simulink library "MIL_Test"  (Simulink 7.0)
values from neighbouring files (symbols this model uses):
  TID = min('TI' == AFT(1:2))    [PAS_callback.m]    (also in PSTID_callback.m = [block '/TID'])
undefined symbols (not defined in the file or in its folder): getdatatypespecs, slcm, StepSize
libraries: simulink x71, MIL_Test x6
(part 3 of 11)

== system MIL_Test/Validation Function/TODO/Validation FunctionsTemplate ==
  InOut Bus : Inport  OutDataType=sfix(16)  OutScaling=2^0
  Arbitration : Subsystem
  Bus Creator : BusCreator  Inputs=2
  Bus Creator4 : BusCreator  Inputs=2
  Bus Selector : BusSelector  OutputSignals=signal1.signal1
  Datatype conversion : Subsystem  TreatAsAtomicUnit=on
  Requirement : Subsystem  mask{No=1}
      mask prompts: No "Number of single Validation Functions"
      mask StyleString: popup(1|2|3|4|5|6|7|8|9|10|11|12|13|14|15|16|17|18|19|20)
      mask CallbackString: ReqInVF_callback(gcb);
  Requirement2 : Subsystem  mask{No=1}
      mask prompts: No "Number of single Validation Functions"
      mask StyleString: popup(1|2|3|4|5|6|7|8|9|10|11|12|13|14|15|16|17|18|19|20)
      mask CallbackString: ReqInVF_callback(gcb);
  Terminator : Terminator
  ReqVerdict Bus : Outport  OutDataType=sfix(16)  OutScaling=2^0
  Overall Verdict : Outport  Port=2  OutDataType=sfix(16)  OutScaling=2^0
  wires:
  Bus Selector/1 -> Arbitration/1(In1), Bus Creator4/1  "<signal1>"
  Bus Creator4/1 -> ReqVerdict Bus/1
  Datatype conversion/1(InOut Bus) -> Requirement/1(InOut Bus), Requirement2/1(InOut Bus)
  Arbitration/1(Out1) -> Overall Verdict/1
  Requirement/1(Validation Information) -> Bus Creator/1
  Bus Creator/1 -> Terminator/1, Bus Selector/1
  InOut Bus/1 -> Datatype conversion/1(InOutBus)
  Requirement2/1(Validation Information) -> Bus Creator/2

== system MIL_Test/Validation Function/Test Evaluation Architecture/<system name> ==
  InOut  Bus : Inport  OutDataType=sfix(16)  OutScaling=2^0
  <Requirement name> : Subsystem  Description=Requirement template. Create a new requirement from this template.  mask{No=1}
      mask prompts: No "Number of single Validation Functions"
      mask StyleString: popup(1|2|3|4|5|6|7|8|9|10|11|12|13|14|15|16|17|18|19|20)
      mask CallbackString: ReqName_callback(gcb);
  Arbitration : Subsystem
  Bus Creator : BusCreator  Inputs=1
  Bus Creator1 : BusCreator  Inputs=2
  Bus Creator4 : BusCreator  Inputs=1
  Bus Selector : BusSelector  OutputSignals=signal1.signal1.signal1
  Signal Conversion : SignalConversion  ConversionOutput=Bus copy
  Terminator : Terminator
  Eval Results : Outport  OutDataType=sfix(16)  OutScaling=2^0
  wires:
  Bus Selector/1 -> Bus Creator4/1, Arbitration/1(In1)  "<signal1>"
  Arbitration/1(Out1) -> Bus Creator1/1
  <Requirement name>/1(Test Info) -> Bus Creator/1
  InOut  Bus/1 -> Signal Conversion/1
  Bus Creator/1 -> Bus Selector/1, Terminator/1
  Signal Conversion/1 -> <Requirement name>/1(InOut Bus)
  Bus Creator4/1 -> Bus Creator1/2
  Bus Creator1/1 -> Eval Results/1

== system MIL_Test/Validation Function/Test Evaluation Architecture/Alternative ==
  InOut Bus : Inport  OutDataType=sfix(16)  OutScaling=2^0
  Alternative Arbitration : Stateflow chart
  Assertions : MIL_Test/Validation Function/Validation FunctionsTemplate/Requirement/Assertions
  Assertions1 : MIL_Test/Validation Function/Validation FunctionsTemplate/Requirement/Assertions
  Assertions2 : MIL_Test/Validation Function/Validation FunctionsTemplate/Requirement/Assertions
  Preconditions : MIL_Test/Validation Function/Validation FunctionsTemplate/Requirement/Preconditions
  Alternative OverallVerdict : Outport  OutDataType=sfix(16)  OutScaling=2^0
  wires:
  Preconditions/1 -> Assertions/1, Assertions1/1, Assertions2/1
  InOut Bus/1 -> Preconditions/1, Assertions/2, Assertions1/2, Assertions2/2
  Assertions/1 -> Alternative Arbitration/1(LocalVerdict1)
  Assertions1/1 -> Alternative Arbitration/2(LocalVerdict2)
  Assertions2/1 -> Alternative Arbitration/3(LocalVerdict3)
  Alternative Arbitration/1(OverallVerdict) -> Alternative OverallVerdict/1

== system MIL_Test/Test Control/Test Control Architecture/Connection Helpers/TestControl for  TestCases Sequencing ==

== system MIL_Test/Test Control/Test Control Architecture/Connection Helpers/TestControl for  TestCases Sequencing NoMask ==
  @StopTime1 : Inport  OutDataType=sfix(16)  OutScaling=2^0
  @[t1,t2]1 : Inport  Port=2  OutDataType=sfix(16)  OutScaling=2^0
  @Time1 : Inport  Port=3  OutDataType=sfix(16)  OutScaling=2^0
  FulfillmentAtTime 2 : ToWorkspace  VariableName=FulfillmentAtTime1  SampleTime=-1  SaveFormat=Structure With Time
  FulfillmentAtTime1 : Display
  FulfillmentDuring 1 : ToWorkspace  VariableName=FulfillmentDuring1  SampleTime=-1  SaveFormat=Structure With Time
  FulfillmentDuring1 : Display
  FulfillmentStopTime 1 : ToWorkspace  VariableName=FulfillmentStopTime1  SampleTime=-1  SaveFormat=Structure With Time
  FulfillmentStopTime1 : Display
  IF Signal@SimStopTime for TC = value1 : Subsystem  mask(Check if Incoming Signal has an Expected Value @ Simulation Stop Time){currentStopTime=on, condition=0}
      mask prompts: currentStopTime "Check @ End of Simulation"; condition "Signal should equal to"
      mask help:
      | The Subsystem checks if the incoming signal (i.e. Overall Verdict, single Requirement Local Verdict, or SUT Outputs) has an expected value at the end of simulation of a previously specified testcase.
      | ____________________________________________________________________
      | 'Check @ End of Simulation' gets the simulation stop time from the window in Simulink.
      | 'Signal should equal to:' is used for giving the condition for the value of signal (i.e.):
      | 2 = none
      | 1 = pass
      | 0 = fail
      | X = anyNumber
      | The subsystem outputs 1 if the condition is fullfilled.
      mask init:
      | % p=get_param(gcb, 'PortHandles');
      | % l=get_param(p.Inport, 'Line'); 
      | % Inp=get_param(p.Inport, 'Name');
      | % set_param(Inp, 'Name', get_param(l, 'Name'));
      mask CallbackString:
      | block = gcb;
      | TCtblock = get_param(get_param(block, 'Parent'), 'Parent');
      | currentStopTime = get_param(TCtblock, 'StopTime');|
  "IF signal @[timeUp, timeDown] for TC = value1" : Subsystem  mask(Check if Incoming Signal has an Expected Value in the given Period of Time){timeDown=11, timeUp=155, condition=1}
      mask prompts: timeDown "Check @ Time from:"; timeUp "Check @ Time till:"; condition "Signal should equal to:"
      mask help:
      | The Subsystem checks if the incoming signal (i.e. Overall Verdict, single Requirement Local Verdict, or SUT Outputs) has an expected value in the given period of time of a previously specified testcase.
      | ____________________________________________________________________
      | 'Check @ Time from:' means the time where the check should begin.
      | 'Check @ Time till:' means the time where the check should end.
      | Constraint: TimeUp > TimeDown.
      | 'Signal should equal to:' is used for giving the condition for the value of signal (i.e.):
      | 2 = none
      | 1 = pass
      | 0 = fail
      | X = anyNumber
      | The subsystem outputs 1 if the condition is fullfilled.
      mask init:
      | % p=get_param(gcb, 'PortHandles');
      | % l=get_param(p.Inport, 'Line'); 
      | % Inp=get_param(p.Inport, 'Name');
      | % set_param(Inp, 'Name', get_param(l, 'Name'));
      mask CallbackString: timeDown = str2double(get_param(gcb,'timeDown'));|timeUp = str2double(get_param(gcb,'timeUp'));|
  IF signal@time for TC = value1 : Subsystem  mask(Check if Incoming Signal has an Expected Value @ given Time){time=22, condition=1}
      mask prompts: time "Check @ Time t"; condition "Signal should equal to"
      mask help:
      | The Subsystem checks if the incoming signal (i.e. Overall Verdict, single Requirement Local Verdict, or SUT Outputs) has an expected value at given time of a previously specified testcase.
      | ____________________________________________________________________
      | 'Check @ Time t' means the time point when the condition should be checked.
      | 'Signal should equal to:' is used for giving the condition for the value of signal (i.e.):
      | 2 = none
      | 1 = pass
      | 0 = fail
      | X = anyNumber
      | The subsystem outputs 1 if the condition is fullfilled.
      mask CallbackString: time = str2double(get_param(gcb,'time'));|
  wires:
  IF signal@time for TC = value1/1(Fulfillment) -> FulfillmentAtTime 2/1, FulfillmentAtTime1/1
  @Time1/1 -> IF signal@time for TC = value1/1(Signal)
  "IF signal @[timeUp, timeDown] for TC = value1"/1(Fulfillment) -> FulfillmentDuring 1/1, FulfillmentDuring1/1
  @[t1,t2]1/1 -> "IF signal @[timeUp, timeDown] for TC = value1"/1(Signal)
  IF Signal@SimStopTime for TC = value1/1(Fulfillment) -> FulfillmentStopTime 1/1, FulfillmentStopTime1/1
  @StopTime1/1 -> IF Signal@SimStopTime for TC = value1/1(Signal)

== system MIL_Test/Test Control/Test Control Architecture/Connection Helpers/TestControl for  TestCases SequencingTemplate ==

== system MIL_Test/Test Control/Test Control Architecture/Test Control  depending on Verdict/Counter ==
  In1 : Inport  OutDataType=sfix(16)  OutScaling=2^0
  Trigger : TriggerPort
  " 1" : DataTypeConversion  Orientation=down  OutDataType=sfix(16)  OutScaling=2^0
  Add : Sum  OutDataType=sfix(16)  OutScaling=2^-10
  Memory : Memory  Orientation=left  InheritSampleTime=on
  Number of triggers : Constant  Value=2  OutDataType=sfix(16)  OutScaling=2^0
  Relational Operator1 : RelationalOperator  Operator===  LogicOutDataTypeMode=boolean
  Scope1 : Scope  NumInputPorts=4
      settings: YMin=182.932~-5~-5~-5  YMax=202.188~5~5~5  SaveName=ScopeData14  MaxDataPoints=5000000
  Out1 : Outport  OutDataType=sfix(16)  OutScaling=2^0
  wires:
  In1/1 -> Add/1, Scope1/2
  Number of triggers/1 -> Relational Operator1/2
  Relational Operator1/1 -> Out1/1
  Add/1 -> " 1"/1, Relational Operator1/1, Scope1/3
  Memory/1 -> Add/2
  " 1"/1 -> Memory/1

== system MIL_Test/Test Control/Test Control Architecture/Test Control Conditions/IF Signal@SimStopTime for TC = value1 ==
  Signal : Inport  OutDataType=sfix(16)  OutScaling=2^0
  Current Sim StopTime : Constant  Value=currentStopTime  OutDataType=sfix(16)  OutScaling=2^0
  If : If  IfExpression=u1 ~= 1
  Model Info : simulink/Model-Wide Utilities/Model Info  SystemSampleTime=-1  InitialBlockCM=None  BlockCM=None  Frame=on  DisplayStringWithTags=|  HorizontalTextAlignment=Center  LeftAlignmentValue=0.5  SourceBlockDiagram=MIL_Test  TagMaxNumber=20
      | Flag Fullfillment = 1, then condition is true 
      | Flag Fullfillment = 0, then condition is false
  if Signal@t for TC = pass : Subsystem
  "if false, then  TC4 for 200" : Subsystem
  "if true, then  TC2 for 400" : Subsystem
  Fulfillment : Outport  OutDataType=sfix(16)  OutScaling=2^0
  wires:
  if Signal@t for TC = pass/1(Control Seq1) -> Fulfillment/1
  If/2 -> "if true, then  TC2 for 400"/Action
  If/1 -> "if false, then  TC4 for 200"/Action
  Signal/1 -> if Signal@t for TC = pass/2(Signal1)
  Current Sim StopTime/1 -> if Signal@t for TC = pass/1(@time)

== system MIL_Test/Test Control/Test Control Architecture/Test Control Conditions/IF signal @[timeUp, timeDown] for TC = value1 ==
  Signal : Inport  OutDataType=sfix(16)  OutScaling=2^0
  TimeDown : Constant  Value=timeDown  OutDataType=sfix(16)  OutScaling=2^0
  TimeUp : Constant  Value=timeUp  OutDataType=sfix(16)  OutScaling=2^0
  if Signal@ [TDown,TUp]  for TC = Value : Subsystem
  Fulfillment : Outport  OutDataType=sfix(16)  OutScaling=2^0
  wires:
  if Signal@ [TDown,TUp]  for TC = Value/1(Control Seq) -> Fulfillment/1
  Signal/1 -> if Signal@ [TDown,TUp]  for TC = Value/3(Signal)
  TimeUp/1 -> if Signal@ [TDown,TUp]  for TC = Value/2(@timeUp)
  TimeDown/1 -> if Signal@ [TDown,TUp]  for TC = Value/1(@timeDown)

== system MIL_Test/Test Control/Test Control Architecture/Test Control Conditions/IF signal@time for TC = value1 ==
  Signal : Inport  OutDataType=sfix(16)  OutScaling=2^0
  given Time : Constant  Value=time  OutDataType=sfix(16)  OutScaling=2^0
  if Signal@t for TC = pass : Subsystem
  Fulfillment : Outport  OutDataType=sfix(16)  OutScaling=2^0
  wires:
  if Signal@t for TC = pass/1(Control Seq) -> Fulfillment/1
  Signal/1 -> if Signal@t for TC = pass/2(Signal1)
  given Time/1 -> if Signal@t for TC = pass/1(@time)

== system MIL_Test/Test Control/Test Control Architecture/Test Control Conditions/IF signal@time1 ==
  Signal : Inport  OutDataType=sfix(16)  OutScaling=2^0
  Current Sim StopTime : Constant  Value=currentStopTime  OutDataType=sfix(16)  OutScaling=2^0
  If : If  IfExpression=u1 ~= 1
  Memory : Memory  Orientation=left
  Model Info : simulink/Model-Wide Utilities/Model Info  SystemSampleTime=-1  InitialBlockCM=None  BlockCM=None  Frame=on  DisplayStringWithTags=|  HorizontalTextAlignment=Center  LeftAlignmentValue=0.5  SourceBlockDiagram=MIL_Test  TagMaxNumber=20
      | Flag Fullfillment = 1, then condition is true 
      | Flag Fullfillment = 0, then condition is false
  if Signal@t for TC = pass : Subsystem
  "if false, then  TC4 for 200" : Subsystem
  "if true, then  TC2 for 400" : Subsystem
  Fulfillment : Outport  OutDataType=sfix(16)  OutScaling=2^0
  wires:
  if Signal@t for TC = pass/1(Control Seq) -> Fulfillment/1
  If/2 -> "if true, then  TC2 for 400"/Action
  If/1 -> "if false, then  TC4 for 200"/Action
  Signal/1 -> if Signal@t for TC = pass/2(Signal1)
  Current Sim StopTime/1 -> if Signal@t for TC = pass/1(@time)

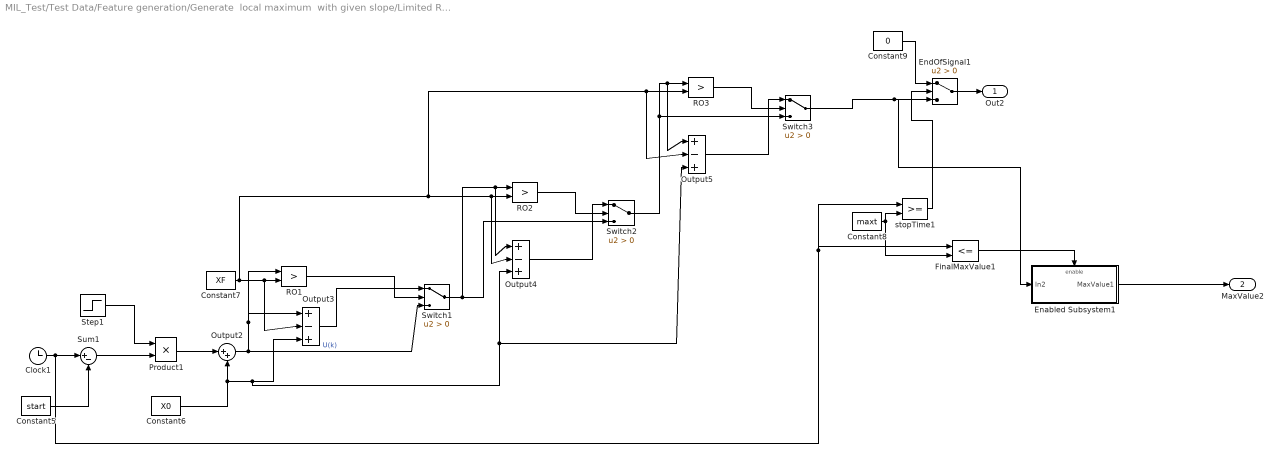
== system MIL_Test/Test Data/Feature generation/Generate  local maximum  with given slope/Limited Ramp Increasing ==
  Clock1 : Clock
      settings: DisableCoverage=on  Decimation=10
  Constant5 : Constant  DisableCoverage=on  Value=start  OutDataType=sfix(16)  OutScaling=2^0
  Constant6 : Constant  DisableCoverage=on  Value=X0  OutDataType=sfix(16)  OutScaling=2^0
  Constant7 : Constant  DisableCoverage=on  Value=XF  OutDataType=sfix(16)  OutScaling=2^0
  Constant8 : Constant  DisableCoverage=on  Value=maxt  OutDataType=sfix(16)  OutScaling=2^0
  Constant9 : Constant  DisableCoverage=on  Value=0  OutDataType=sfix(16)  OutScaling=2^0
  Enabled Subsystem1 : Subsystem  TreatAsAtomicUnit=on
  EndOfSignal1 : Switch  Criteria=u2 > Threshold
  FinalMaxValue1 : RelationalOperator  Operator=<=  LogicOutDataTypeMode=boolean
  Output2 : Sum  Inputs=|++  OutDataType=sfix(16)  OutScaling=2^0  SaturateOnIntegerOverflow=on  InputSameDT=on
  Output3 : Sum  Inputs=|+-+  OutDataType=sfix(16)  OutScaling=2^0  SaturateOnIntegerOverflow=on  InputSameDT=on
  Output4 : Sum  Inputs=|+-+  OutDataType=sfix(16)  OutScaling=2^0  SaturateOnIntegerOverflow=on  InputSameDT=on
  Output5 : Sum  Inputs=|+-+  OutDataType=sfix(16)  OutScaling=2^0  SaturateOnIntegerOverflow=on  InputSameDT=on
  Product1 : Product  DisableCoverage=on  OutDataType=sfix(16)  OutScaling=2^0  SaturateOnIntegerOverflow=on  InputSameDT=on
  RO1 : RelationalOperator  Operator=>  LogicOutDataTypeMode=boolean
  RO2 : RelationalOperator  Operator=>  LogicOutDataTypeMode=boolean
  RO3 : RelationalOperator  Operator=>  LogicOutDataTypeMode=boolean
  Step1 : Step  DisableCoverage=on  Time=start  After=slope  SampleTime=0
  Sum1 : Sum  DisableCoverage=on  Inputs=|+-  OutDataType=sfix(16)  OutScaling=2^0  SaturateOnIntegerOverflow=on  InputSameDT=on
  Switch1 : Switch  Criteria=u2 > Threshold
  Switch2 : Switch  Criteria=u2 > Threshold
  Switch3 : Switch  Criteria=u2 > Threshold
  stopTime1 : RelationalOperator  LogicOutDataTypeMode=boolean
  Out2 : Outport  OutDataType=sfix(16)  OutScaling=2^0
  MaxValue2 : Outport  Port=2  OutDataType=sfix(16)  OutScaling=2^0
  wires:
  Enabled Subsystem1/1(MaxValue1) -> MaxValue2/1
  FinalMaxValue1/1 -> Enabled Subsystem1/Enable
  EndOfSignal1/1 -> Out2/1
  Constant9/1 -> EndOfSignal1/1
  stopTime1/1 -> EndOfSignal1/2
  Constant8/1 -> FinalMaxValue1/2, stopTime1/2
  RO1/1 -> Switch1/2
  Output3/1 -> Switch1/1
  Output2/1 -> Switch1/3, RO1/1, Output3/1  "U(k)"
  Output5/1 -> Switch3/1
  RO3/1 -> Switch3/2
  Switch3/1 -> Enabled Subsystem1/1(In2), EndOfSignal1/3
  Switch2/1 -> Output5/1, RO3/1, Switch3/3
  Output4/1 -> Switch2/1
  RO2/1 -> Switch2/2
  Switch1/1 -> Output4/1, RO2/1, Switch2/3
  Constant7/1 -> Output5/2, RO3/2, Output4/2, RO2/2, Output3/2, RO1/2
  Clock1/1 -> stopTime1/1, FinalMaxValue1/1, Sum1/1
  Constant5/1 -> Sum1/2
  Sum1/1 -> Product1/2
  Constant6/1 -> Output5/3, Output4/3, Output3/3, Output2/2
  Product1/1 -> Output2/1
  Step1/1 -> Product1/1

== system MIL_Test/Test Data/Feature generation/Generate  local maximum  with given slope/Limited Ramp  Decreasing1 ==
  InitialValue : Inport  OutDataType=sfix(16)  OutScaling=2^0
  Clock : Clock
      settings: DisableCoverage=on  Decimation=10
  Constant : Constant  DisableCoverage=on  Value=maxt  OutDataType=sfix(16)  OutScaling=2^0
  Constant4 : Constant  DisableCoverage=on  Value=0  OutDataType=sfix(16)  OutScaling=2^0
  NoStartOfSignal : Switch  Criteria=u2 > Threshold
  NotYetStartTime : RelationalOperator  Operator=<  LogicOutDataTypeMode=boolean
  Output : Sum  Inputs=|++  OutDataType=sfix(16)  OutScaling=2^0  SaturateOnIntegerOverflow=on  InputSameDT=on
  Product : Product  DisableCoverage=on  OutDataType=sfix(16)  OutScaling=2^0  SaturateOnIntegerOverflow=on  InputSameDT=on
  Step : Step  DisableCoverage=on  Time=maxt  After=-slope  SampleTime=0
  Sum : Sum  DisableCoverage=on  Inputs=|+-  OutDataType=sfix(16)  OutScaling=2^0  SaturateOnIntegerOverflow=on  InputSameDT=on
  Out1 : Outport  OutDataType=sfix(16)  OutScaling=2^0
  wires:
  NoStartOfSignal/1 -> Out1/1
  Constant4/1 -> NoStartOfSignal/1
  NotYetStartTime/1 -> NoStartOfSignal/2
  Step/1 -> Product/1
  Product/1 -> Output/1
  InitialValue/1 -> Output/2
  Output/1 -> NoStartOfSignal/3
  Sum/1 -> Product/2
  Constant/1 -> NotYetStartTime/2, Sum/2
  Clock/1 -> NotYetStartTime/1, Sum/1

== system MIL_Test/Test Data/Feature generation/Generate complete step/Hold Time ==
  Clock : Inport  OutDataType=sfix(16)  OutScaling=2^0
  Enable : EnablePort
  Write : DataStoreWrite  DataStoreName=triggerTime  SampleTime=-1
  wires:
  Clock/1 -> Write/1

== system MIL_Test/Test Data/Feature generation/Generate complete step/Hold Value ==
  In1 : Inport  OutDataType=sfix(16)  OutScaling=2^0
  Enable : EnablePort
  v_Des : Outport  OutDataType=sfix(16)  OutScaling=2^0
  wires:
  In1/1 -> v_Des/1

== system MIL_Test/Test Data/Feature generation/Generate timed constant/Repeating Sequence ==
  Clock : Clock
      settings: Decimation=10
  Fcn1 : Fcn  Expr=rem(u[1],period)
  Look-Up Table1 : Lookup  InputValues=rep_seq_t - min(rep_seq_t)  Table=rep_seq_y  OutDataType=sfix(16)  OutScaling=2^0  SaturateOnIntegerOverflow=on
  Output : SignalConversion  ConversionOutput=Contiguous copy
  Sum : Sum  Inputs=+-  OutDataType=sfix(16)  OutScaling=2^0  SaturateOnIntegerOverflow=on  InputSameDT=on
  startTime : S-Function  FunctionName=sfun_tstart
  Out1 : Outport  OutDataType=sfix(16)  OutScaling=2^0
  wires:
  Fcn1/1 -> Look-Up Table1/1
  Sum/1 -> Fcn1/1
  Clock/1 -> Sum/1
  startTime/1 -> Sum/2
  Look-Up Table1/1 -> Output/1
  Output/1 -> Out1/1

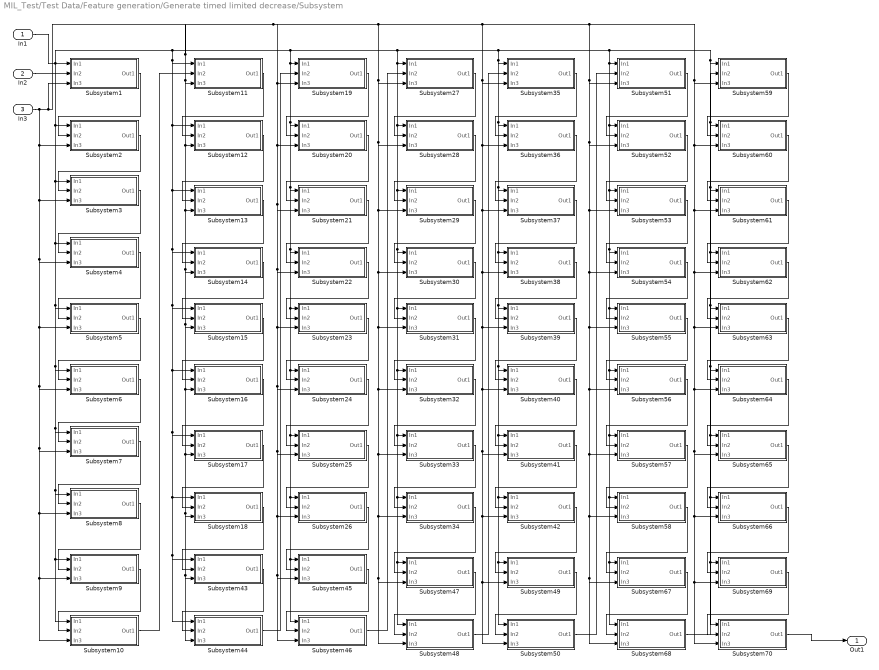
== system MIL_Test/Test Data/Feature generation/Generate timed limited decrease/Subsystem ==
  In1 : Inport  OutDataType=sfix(16)  OutScaling=2^0
  In2 : Inport  Port=2  OutDataType=sfix(16)  OutScaling=2^0
  In3 : Inport  Port=3  OutDataType=sfix(16)  OutScaling=2^0
  Subsystem1 : Subsystem
  Subsystem10 : Subsystem
  Subsystem11 : Subsystem
  Subsystem12 : Subsystem
  Subsystem13 : Subsystem
  Subsystem14 : Subsystem
  Subsystem15 : Subsystem
  Subsystem16 : Subsystem
  Subsystem17 : Subsystem
  Subsystem18 : Subsystem
  Subsystem19 : Subsystem
  Subsystem2 : Subsystem
  Subsystem20 : Subsystem
  Subsystem21 : Subsystem
  Subsystem22 : Subsystem
  Subsystem23 : Subsystem
  Subsystem24 : Subsystem
  Subsystem25 : Subsystem
  Subsystem26 : Subsystem
  Subsystem27 : Subsystem
  Subsystem28 : Subsystem
  Subsystem29 : Subsystem
  Subsystem3 : Subsystem
  Subsystem30 : Subsystem
  Subsystem31 : Subsystem
  Subsystem32 : Subsystem
  Subsystem33 : Subsystem
  Subsystem34 : Subsystem
  Subsystem35 : Subsystem
  Subsystem36 : Subsystem
  Subsystem37 : Subsystem
  Subsystem38 : Subsystem
  Subsystem39 : Subsystem
  Subsystem4 : Subsystem
  Subsystem40 : Subsystem
  Subsystem41 : Subsystem
  Subsystem42 : Subsystem
  Subsystem43 : Subsystem
  Subsystem44 : Subsystem
  Subsystem45 : Subsystem
  Subsystem46 : Subsystem
  Subsystem47 : Subsystem
  Subsystem48 : Subsystem
  Subsystem49 : Subsystem
  Subsystem5 : Subsystem
  Subsystem50 : Subsystem
  Subsystem51 : Subsystem
  Subsystem52 : Subsystem
  Subsystem53 : Subsystem
  Subsystem54 : Subsystem
  Subsystem55 : Subsystem
  Subsystem56 : Subsystem
  Subsystem57 : Subsystem
  Subsystem58 : Subsystem
  Subsystem59 : Subsystem
  Subsystem6 : Subsystem
  Subsystem60 : Subsystem
  Subsystem61 : Subsystem
  Subsystem62 : Subsystem
  Subsystem63 : Subsystem
  Subsystem64 : Subsystem
  Subsystem65 : Subsystem
  Subsystem66 : Subsystem
  Subsystem67 : Subsystem
  Subsystem68 : Subsystem
  Subsystem69 : Subsystem
  Subsystem7 : Subsystem
  Subsystem70 : Subsystem
  Subsystem8 : Subsystem
  Subsystem9 : Subsystem
  Out1 : Outport  OutDataType=sfix(16)  OutScaling=2^0
  wires:
  In1/1 -> Subsystem1/1(In1), Subsystem2/1(In1), Subsystem3/1(In1), Subsystem4/1(In1), Subsystem5/1(In1), Subsystem6/1(In1), Subsystem7/1(In1), Subsystem8/1(In1), Subsystem9/1(In1), Subsystem10/1(In1), Subsystem27/1(In1), Subsystem28/1(In1), Subsystem29/1(In1), Subsystem30/1(In1), Subsystem31/1(In1), Subsystem32/1(In1), Subsystem33/1(In1), Subsystem34/1(In1), Subsystem47/1(In1), Subsystem48/1(In1), Subsystem35/1(In1), Subsystem36/1(In1), Subsystem37/1(In1), Subsystem38/1(In1), Subsystem39/1(In1), Subsystem40/1(In1), Subsystem41/1(In1), Subsystem42/1(In1), Subsystem49/1(In1), Subsystem50/1(In1), Subsystem51/1(In1), Subsystem52/1(In1), Subsystem53/1(In1), Subsystem54/1(In1), Subsystem55/1(In1), Subsystem56/1(In1), Subsystem57/1(In1), Subsystem58/1(In1), Subsystem67/1(In1), Subsystem68/1(In1), Subsystem59/1(In1), Subsystem60/1(In1), Subsystem61/1(In1), Subsystem62/1(In1), Subsystem63/1(In1), Subsystem64/1(In1), Subsystem65/1(In1), Subsystem66/1(In1), Subsystem69/1(In1), Subsystem70/1(In1), Subsystem19/1(In1), Subsystem20/1(In1), Subsystem21/1(In1), Subsystem22/1(In1), Subsystem23/1(In1), Subsystem24/1(In1), Subsystem25/1(In1), Subsystem26/1(In1), Subsystem45/1(In1), Subsystem46/1(In1), Subsystem11/1(In1), Subsystem12/1(In1), Subsystem13/1(In1), Subsystem14/1(In1), Subsystem15/1(In1), Subsystem16/1(In1), Subsystem17/1(In1), Subsystem18/1(In1), Subsystem43/1(In1), Subsystem44/1(In1)
  In2/1 -> Subsystem1/2(In2)
  In3/1 -> Subsystem2/3(In3), Subsystem3/3(In3), Subsystem4/3(In3), Subsystem5/3(In3), Subsystem6/3(In3), Subsystem7/3(In3), Subsystem8/3(In3), Subsystem9/3(In3), Subsystem10/3(In3), Subsystem1/3(In3), Subsystem12/3(In3), Subsystem13/3(In3), Subsystem14/3(In3), Subsystem15/3(In3), Subsystem16/3(In3), Subsystem17/3(In3), Subsystem18/3(In3), Subsystem43/3(In3), Subsystem44/3(In3), Subsystem11/3(In3), Subsystem19/3(In3), Subsystem20/3(In3), Subsystem21/3(In3), Subsystem22/3(In3), Subsystem23/3(In3), Subsystem24/3(In3), Subsystem25/3(In3), Subsystem26/3(In3), Subsystem45/3(In3), Subsystem46/3(In3), Subsystem27/3(In3), Subsystem28/3(In3), Subsystem29/3(In3), Subsystem30/3(In3), Subsystem31/3(In3), Subsystem32/3(In3), Subsystem33/3(In3), Subsystem34/3(In3), Subsystem47/3(In3), Subsystem48/3(In3), Subsystem35/3(In3), Subsystem36/3(In3), Subsystem37/3(In3), Subsystem38/3(In3), Subsystem39/3(In3), Subsystem40/3(In3), Subsystem41/3(In3), Subsystem42/3(In3), Subsystem49/3(In3), Subsystem50/3(In3), Subsystem51/3(In3), Subsystem52/3(In3), Subsystem53/3(In3), Subsystem54/3(In3), Subsystem55/3(In3), Subsystem56/3(In3), Subsystem57/3(In3), Subsystem58/3(In3), Subsystem67/3(In3), Subsystem68/3(In3), Subsystem59/3(In3), Subsystem60/3(In3), Subsystem61/3(In3), Subsystem62/3(In3), Subsystem63/3(In3), Subsystem64/3(In3), Subsystem65/3(In3), Subsystem66/3(In3), Subsystem69/3(In3), Subsystem70/3(In3)
  Subsystem1/1(Out1) -> Subsystem2/2(In2)
  Subsystem2/1(Out1) -> Subsystem3/2(In2)
  Subsystem3/1(Out1) -> Subsystem4/2(In2)
  Subsystem4/1(Out1) -> Subsystem5/2(In2)
  Subsystem5/1(Out1) -> Subsystem6/2(In2)
  Subsystem6/1(Out1) -> Subsystem7/2(In2)
  Subsystem7/1(Out1) -> Subsystem8/2(In2)
  Subsystem8/1(Out1) -> Subsystem9/2(In2)
  Subsystem9/1(Out1) -> Subsystem10/2(In2)
  Subsystem11/1(Out1) -> Subsystem12/2(In2)
  Subsystem12/1(Out1) -> Subsystem13/2(In2)
  Subsystem14/1(Out1) -> Subsystem15/2(In2)
  Subsystem13/1(Out1) -> Subsystem14/2(In2)
  Subsystem15/1(Out1) -> Subsystem16/2(In2)
  Subsystem16/1(Out1) -> Subsystem17/2(In2)
  Subsystem17/1(Out1) -> Subsystem18/2(In2)
  Subsystem10/1(Out1) -> Subsystem11/2(In2)
  Subsystem18/1(Out1) -> Subsystem43/2(In2)
  Subsystem43/1(Out1) -> Subsystem44/2(In2)
  Subsystem19/1(Out1) -> Subsystem20/2(In2)
  Subsystem20/1(Out1) -> Subsystem21/2(In2)
  Subsystem21/1(Out1) -> Subsystem22/2(In2)
  Subsystem22/1(Out1) -> Subsystem23/2(In2)
  Subsystem24/1(Out1) -> Subsystem25/2(In2)
  Subsystem23/1(Out1) -> Subsystem24/2(In2)
  Subsystem25/1(Out1) -> Subsystem26/2(In2)
  Subsystem26/1(Out1) -> Subsystem45/2(In2)
  Subsystem45/1(Out1) -> Subsystem46/2(In2)
  Subsystem27/1(Out1) -> Subsystem28/2(In2)
  Subsystem28/1(Out1) -> Subsystem29/2(In2)
  Subsystem29/1(Out1) -> Subsystem30/2(In2)
  Subsystem30/1(Out1) -> Subsystem31/2(In2)
  Subsystem31/1(Out1) -> Subsystem32/2(In2)
  Subsystem32/1(Out1) -> Subsystem33/2(In2)
  Subsystem33/1(Out1) -> Subsystem34/2(In2)
  Subsystem34/1(Out1) -> Subsystem47/2(In2)
  Subsystem47/1(Out1) -> Subsystem48/2(In2)
  Subsystem35/1(Out1) -> Subsystem36/2(In2)
  Subsystem36/1(Out1) -> Subsystem37/2(In2)
  Subsystem37/1(Out1) -> Subsystem38/2(In2)
  Subsystem38/1(Out1) -> Subsystem39/2(In2)
  Subsystem39/1(Out1) -> Subsystem40/2(In2)
  Subsystem40/1(Out1) -> Subsystem41/2(In2)
  Subsystem41/1(Out1) -> Subsystem42/2(In2)
  Subsystem42/1(Out1) -> Subsystem49/2(In2)
  Subsystem49/1(Out1) -> Subsystem50/2(In2)
  Subsystem44/1(Out1) -> Subsystem19/2(In2)
  Subsystem46/1(Out1) -> Subsystem27/2(In2)
  Subsystem48/1(Out1) -> Subsystem35/2(In2)
  Subsystem51/1(Out1) -> Subsystem52/2(In2)
  Subsystem52/1(Out1) -> Subsystem53/2(In2)
  Subsystem53/1(Out1) -> Subsystem54/2(In2)
  Subsystem54/1(Out1) -> Subsystem55/2(In2)
  Subsystem55/1(Out1) -> Subsystem56/2(In2)
  Subsystem56/1(Out1) -> Subsystem57/2(In2)
  Subsystem57/1(Out1) -> Subsystem58/2(In2)
  Subsystem58/1(Out1) -> Subsystem67/2(In2)
  Subsystem67/1(Out1) -> Subsystem68/2(In2)
  Subsystem59/1(Out1) -> Subsystem60/2(In2)
  Subsystem60/1(Out1) -> Subsystem61/2(In2)
  Subsystem61/1(Out1) -> Subsystem62/2(In2)
  Subsystem62/1(Out1) -> Subsystem63/2(In2)
  Subsystem63/1(Out1) -> Subsystem64/2(In2)
  Subsystem64/1(Out1) -> Subsystem65/2(In2)
  Subsystem65/1(Out1) -> Subsystem66/2(In2)
  Subsystem66/1(Out1) -> Subsystem69/2(In2)
  Subsystem69/1(Out1) -> Subsystem70/2(In2)
  Subsystem50/1(Out1) -> Subsystem51/2(In2)
  Subsystem68/1(Out1) -> Subsystem59/2(In2)
  Subsystem70/1(Out1) -> Out1/1

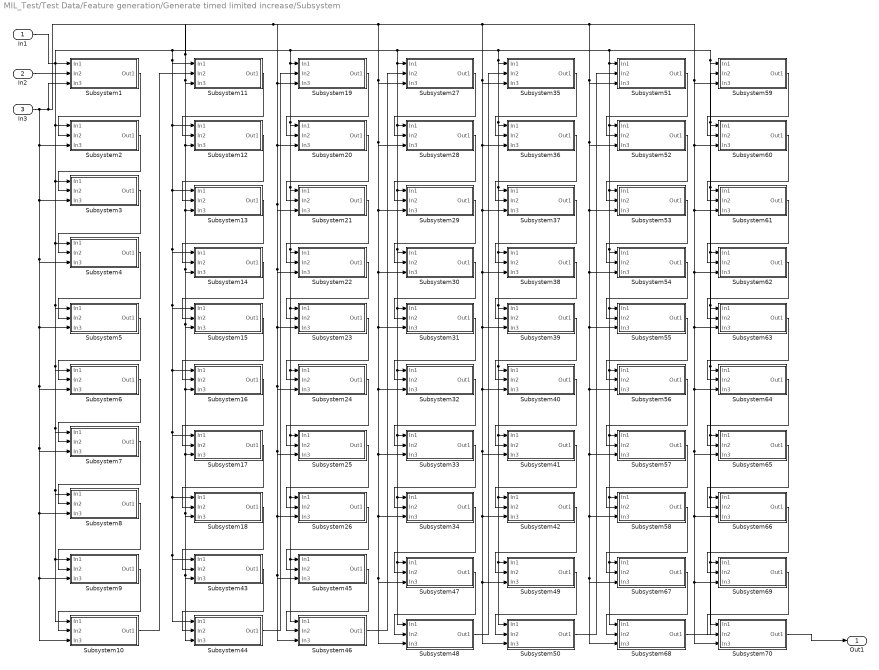
== system MIL_Test/Test Data/Feature generation/Generate timed limited increase/Subsystem ==
  In1 : Inport  OutDataType=sfix(16)  OutScaling=2^0
  In2 : Inport  Port=2  OutDataType=sfix(16)  OutScaling=2^0
  In3 : Inport  Port=3  OutDataType=sfix(16)  OutScaling=2^0
  Subsystem1 : Subsystem
  Subsystem10 : Subsystem
  Subsystem11 : Subsystem
  Subsystem12 : Subsystem
  Subsystem13 : Subsystem
  Subsystem14 : Subsystem
  Subsystem15 : Subsystem
  Subsystem16 : Subsystem
  Subsystem17 : Subsystem
  Subsystem18 : Subsystem
  Subsystem19 : Subsystem
  Subsystem2 : Subsystem
  Subsystem20 : Subsystem
  Subsystem21 : Subsystem
  Subsystem22 : Subsystem
  Subsystem23 : Subsystem
  Subsystem24 : Subsystem
  Subsystem25 : Subsystem
  Subsystem26 : Subsystem
  Subsystem27 : Subsystem
  Subsystem28 : Subsystem
  Subsystem29 : Subsystem
  Subsystem3 : Subsystem
  Subsystem30 : Subsystem
  Subsystem31 : Subsystem
  Subsystem32 : Subsystem
  Subsystem33 : Subsystem
  Subsystem34 : Subsystem
  Subsystem35 : Subsystem
  Subsystem36 : Subsystem
  Subsystem37 : Subsystem
  Subsystem38 : Subsystem
  Subsystem39 : Subsystem
  Subsystem4 : Subsystem
  Subsystem40 : Subsystem
  Subsystem41 : Subsystem
  Subsystem42 : Subsystem
  Subsystem43 : Subsystem
  Subsystem44 : Subsystem
  Subsystem45 : Subsystem
  Subsystem46 : Subsystem
  Subsystem47 : Subsystem
  Subsystem48 : Subsystem
  Subsystem49 : Subsystem
  Subsystem5 : Subsystem
  Subsystem50 : Subsystem
  Subsystem51 : Subsystem
  Subsystem52 : Subsystem
  Subsystem53 : Subsystem
  Subsystem54 : Subsystem
  Subsystem55 : Subsystem
  Subsystem56 : Subsystem
  Subsystem57 : Subsystem
  Subsystem58 : Subsystem
  Subsystem59 : Subsystem
  Subsystem6 : Subsystem
  Subsystem60 : Subsystem
  Subsystem61 : Subsystem
  Subsystem62 : Subsystem
  Subsystem63 : Subsystem
  Subsystem64 : Subsystem
  Subsystem65 : Subsystem
  Subsystem66 : Subsystem
  Subsystem67 : Subsystem
  Subsystem68 : Subsystem
  Subsystem69 : Subsystem
  Subsystem7 : Subsystem
  Subsystem70 : Subsystem
  Subsystem8 : Subsystem
  Subsystem9 : Subsystem
  Out1 : Outport  OutDataType=sfix(16)  OutScaling=2^0
  wires:
  In1/1 -> Subsystem1/1(In1), Subsystem2/1(In1), Subsystem3/1(In1), Subsystem4/1(In1), Subsystem5/1(In1), Subsystem6/1(In1), Subsystem7/1(In1), Subsystem8/1(In1), Subsystem9/1(In1), Subsystem10/1(In1), Subsystem27/1(In1), Subsystem28/1(In1), Subsystem29/1(In1), Subsystem30/1(In1), Subsystem31/1(In1), Subsystem32/1(In1), Subsystem33/1(In1), Subsystem34/1(In1), Subsystem47/1(In1), Subsystem48/1(In1), Subsystem35/1(In1), Subsystem36/1(In1), Subsystem37/1(In1), Subsystem38/1(In1), Subsystem39/1(In1), Subsystem40/1(In1), Subsystem41/1(In1), Subsystem42/1(In1), Subsystem49/1(In1), Subsystem50/1(In1), Subsystem51/1(In1), Subsystem52/1(In1), Subsystem53/1(In1), Subsystem54/1(In1), Subsystem55/1(In1), Subsystem56/1(In1), Subsystem57/1(In1), Subsystem58/1(In1), Subsystem67/1(In1), Subsystem68/1(In1), Subsystem59/1(In1), Subsystem60/1(In1), Subsystem61/1(In1), Subsystem62/1(In1), Subsystem63/1(In1), Subsystem64/1(In1), Subsystem65/1(In1), Subsystem66/1(In1), Subsystem69/1(In1), Subsystem70/1(In1), Subsystem19/1(In1), Subsystem20/1(In1), Subsystem21/1(In1), Subsystem22/1(In1), Subsystem23/1(In1), Subsystem24/1(In1), Subsystem25/1(In1), Subsystem26/1(In1), Subsystem45/1(In1), Subsystem46/1(In1), Subsystem11/1(In1), Subsystem12/1(In1), Subsystem13/1(In1), Subsystem14/1(In1), Subsystem15/1(In1), Subsystem16/1(In1), Subsystem17/1(In1), Subsystem18/1(In1), Subsystem43/1(In1), Subsystem44/1(In1)
  In2/1 -> Subsystem1/2(In2)
  In3/1 -> Subsystem2/3(In3), Subsystem3/3(In3), Subsystem4/3(In3), Subsystem5/3(In3), Subsystem6/3(In3), Subsystem7/3(In3), Subsystem8/3(In3), Subsystem9/3(In3), Subsystem10/3(In3), Subsystem1/3(In3), Subsystem12/3(In3), Subsystem13/3(In3), Subsystem14/3(In3), Subsystem15/3(In3), Subsystem16/3(In3), Subsystem17/3(In3), Subsystem18/3(In3), Subsystem43/3(In3), Subsystem44/3(In3), Subsystem11/3(In3), Subsystem19/3(In3), Subsystem20/3(In3), Subsystem21/3(In3), Subsystem22/3(In3), Subsystem23/3(In3), Subsystem24/3(In3), Subsystem25/3(In3), Subsystem26/3(In3), Subsystem45/3(In3), Subsystem46/3(In3), Subsystem27/3(In3), Subsystem28/3(In3), Subsystem29/3(In3), Subsystem30/3(In3), Subsystem31/3(In3), Subsystem32/3(In3), Subsystem33/3(In3), Subsystem34/3(In3), Subsystem47/3(In3), Subsystem48/3(In3), Subsystem35/3(In3), Subsystem36/3(In3), Subsystem37/3(In3), Subsystem38/3(In3), Subsystem39/3(In3), Subsystem40/3(In3), Subsystem41/3(In3), Subsystem42/3(In3), Subsystem49/3(In3), Subsystem50/3(In3), Subsystem51/3(In3), Subsystem52/3(In3), Subsystem53/3(In3), Subsystem54/3(In3), Subsystem55/3(In3), Subsystem56/3(In3), Subsystem57/3(In3), Subsystem58/3(In3), Subsystem67/3(In3), Subsystem68/3(In3), Subsystem59/3(In3), Subsystem60/3(In3), Subsystem61/3(In3), Subsystem62/3(In3), Subsystem63/3(In3), Subsystem64/3(In3), Subsystem65/3(In3), Subsystem66/3(In3), Subsystem69/3(In3), Subsystem70/3(In3)
  Subsystem1/1(Out1) -> Subsystem2/2(In2)
  Subsystem2/1(Out1) -> Subsystem3/2(In2)
  Subsystem3/1(Out1) -> Subsystem4/2(In2)
  Subsystem4/1(Out1) -> Subsystem5/2(In2)
  Subsystem5/1(Out1) -> Subsystem6/2(In2)
  Subsystem6/1(Out1) -> Subsystem7/2(In2)
  Subsystem7/1(Out1) -> Subsystem8/2(In2)
  Subsystem8/1(Out1) -> Subsystem9/2(In2)
  Subsystem9/1(Out1) -> Subsystem10/2(In2)
  Subsystem11/1(Out1) -> Subsystem12/2(In2)
  Subsystem12/1(Out1) -> Subsystem13/2(In2)
  Subsystem14/1(Out1) -> Subsystem15/2(In2)
  Subsystem13/1(Out1) -> Subsystem14/2(In2)
  Subsystem15/1(Out1) -> Subsystem16/2(In2)
  Subsystem16/1(Out1) -> Subsystem17/2(In2)
  Subsystem17/1(Out1) -> Subsystem18/2(In2)
  Subsystem10/1(Out1) -> Subsystem11/2(In2)
  Subsystem18/1(Out1) -> Subsystem43/2(In2)
  Subsystem43/1(Out1) -> Subsystem44/2(In2)
  Subsystem19/1(Out1) -> Subsystem20/2(In2)
  Subsystem20/1(Out1) -> Subsystem21/2(In2)
  Subsystem21/1(Out1) -> Subsystem22/2(In2)
  Subsystem22/1(Out1) -> Subsystem23/2(In2)
  Subsystem24/1(Out1) -> Subsystem25/2(In2)
  Subsystem23/1(Out1) -> Subsystem24/2(In2)
  Subsystem25/1(Out1) -> Subsystem26/2(In2)
  Subsystem26/1(Out1) -> Subsystem45/2(In2)
  Subsystem45/1(Out1) -> Subsystem46/2(In2)
  Subsystem27/1(Out1) -> Subsystem28/2(In2)
  Subsystem28/1(Out1) -> Subsystem29/2(In2)
  Subsystem29/1(Out1) -> Subsystem30/2(In2)
  Subsystem30/1(Out1) -> Subsystem31/2(In2)
  Subsystem31/1(Out1) -> Subsystem32/2(In2)
  Subsystem32/1(Out1) -> Subsystem33/2(In2)
  Subsystem33/1(Out1) -> Subsystem34/2(In2)
  Subsystem34/1(Out1) -> Subsystem47/2(In2)
  Subsystem47/1(Out1) -> Subsystem48/2(In2)
  Subsystem35/1(Out1) -> Subsystem36/2(In2)
  Subsystem36/1(Out1) -> Subsystem37/2(In2)
  Subsystem37/1(Out1) -> Subsystem38/2(In2)
  Subsystem38/1(Out1) -> Subsystem39/2(In2)
  Subsystem39/1(Out1) -> Subsystem40/2(In2)
  Subsystem40/1(Out1) -> Subsystem41/2(In2)
  Subsystem41/1(Out1) -> Subsystem42/2(In2)
  Subsystem42/1(Out1) -> Subsystem49/2(In2)
  Subsystem49/1(Out1) -> Subsystem50/2(In2)
  Subsystem44/1(Out1) -> Subsystem19/2(In2)
  Subsystem46/1(Out1) -> Subsystem27/2(In2)
  Subsystem48/1(Out1) -> Subsystem35/2(In2)
  Subsystem51/1(Out1) -> Subsystem52/2(In2)
  Subsystem52/1(Out1) -> Subsystem53/2(In2)
  Subsystem53/1(Out1) -> Subsystem54/2(In2)
  Subsystem54/1(Out1) -> Subsystem55/2(In2)
  Subsystem55/1(Out1) -> Subsystem56/2(In2)
  Subsystem56/1(Out1) -> Subsystem57/2(In2)
  Subsystem57/1(Out1) -> Subsystem58/2(In2)
  Subsystem58/1(Out1) -> Subsystem67/2(In2)
  Subsystem67/1(Out1) -> Subsystem68/2(In2)
  Subsystem59/1(Out1) -> Subsystem60/2(In2)
  Subsystem60/1(Out1) -> Subsystem61/2(In2)
  Subsystem61/1(Out1) -> Subsystem62/2(In2)
  Subsystem62/1(Out1) -> Subsystem63/2(In2)
  Subsystem63/1(Out1) -> Subsystem64/2(In2)
  Subsystem64/1(Out1) -> Subsystem65/2(In2)
  Subsystem65/1(Out1) -> Subsystem66/2(In2)
  Subsystem66/1(Out1) -> Subsystem69/2(In2)
  Subsystem69/1(Out1) -> Subsystem70/2(In2)
  Subsystem50/1(Out1) -> Subsystem51/2(In2)
  Subsystem68/1(Out1) -> Subsystem59/2(In2)
  Subsystem70/1(Out1) -> Out1/1

== system MIL_Test/Test Data/Test Data Architecture/<Test data generator>/<Requirement name> ==
  Out Bus : Inport  OutDataType=sfix(16)  OutScaling=2^0
  <Preconditions name> : Subsystem
  Initialisation & Stabilisation : Subsystem
  Sequencing of test data in time due to Preconditions : Stateflow chart
  switch <signal1> : MultiPortSwitch  Inputs=2
  <signal1> : Outport  OutDataType=sfix(16)  OutScaling=2^0
  wires:
  Initialisation & Stabilisation/1(<signal1>) -> switch <signal1>/3
  <Preconditions name>/2(<signal1>) -> switch <signal1>/2
  Sequencing of test data in time due to Preconditions/1(TDPre) -> switch <signal1>/1
  <Preconditions name>/1(Activate) -> Sequencing of test data in time due to Preconditions/1(Activate)
  switch <signal1>/1 -> <signal1>/1
  Out Bus/1 -> <Preconditions name>/1(Out Bus)

== system MIL_Test/Validation Function/Feature extraction/Complete step detection/Step detection ==
  R : Inport  OutDataType=sfix(16)  OutScaling=2^0
  Step : Inport  Port=2  OutDataType=sfix(16)  OutScaling=2^0
  Step response : Inport  Port=3  OutDataType=sfix(16)  OutScaling=2^0
  Active if signals constant for some specified time : Subsystem
  Detect constant : Subsystem  TreatAsAtomicUnit=on  mask(Feature extraction block){RT=0.0001}
      mask prompts: RT "Relative tolerance in %"
      mask help: Detect if the signal value is constant (using the last two signal values) allowing for a user-defined relative deviation
      mask CallbackString:
      | if or( (str2double(get_param(gcb,'RT')) < 0), (str2double(get_param(gcb,'RT')) > 100))
      |     error(['Relative tolerance value (' get_param(gcb,'RT') ') out of range. Please give a value between 0 and 100.']);
      | else
      |     set_param([gcb '/Relative tolerance/Relative Tolerance'],'Value',get_param(gcb,'RT'));
      | end
  Detect decrease : Subsystem  TreatAsAtomicUnit=on  mask(Detect increase){Param=0}
      mask prompts: Param "Mask Parameter 1:"
  Detect increase : Subsystem  TreatAsAtomicUnit=on  mask(Detect increase){Param=0}
      mask prompts: Param "Mask Parameter 1:"
  Detect increase2 : Subsystem  TreatAsAtomicUnit=on  mask(Detect increase){Param=0}
      mask prompts: Param "Mask Parameter 1:"
  Hold1 : Subsystem  TreatAsAtomicUnit=on
      mask Display: patch(-0.31+[0.4 0.46 0.46 0.54 0.54 0.6 0.6 0.55 0.55 0.45 0.45 0.4],-0.19+[0.85 0.85 0.95 0.95 0.85 0.85 0.87 0.87 0.96 0.96 0.87 0.87],[0 0 0]);
  Logical Operator : Logic  AllPortsSameDT=off  OutDataTypeMode=boolean
  Logical Operator1 : Logic  Operator=NOT  AllPortsSameDT=off  OutDataTypeMode=boolean
  Logical Operator2 : Logic  Operator=OR  Inputs=3  AllPortsSameDT=off  OutDataTypeMode=boolean
  Memory2 : Memory
  End of complete step : Outport  OutDataType=sfix(16)  OutScaling=2^0
  wires:
  Detect increase/1(Increase) -> Logical Operator2/1
  Detect constant/1(Constant) -> Logical Operator1/1
  Detect decrease/1(Decrease) -> Logical Operator2/2
  Logical Operator2/1 -> Hold1/1(" ")
  R/1 -> Hold1/2("    ")
  Step/1 -> Active if signals constant for some specified time/1(Signal1), Detect constant/1(Signal)
  Step response/1 -> Active if signals constant for some specified time/2(Signal 2)
  Active if signals constant for some specified time/1(Constant signals) -> Detect decrease/1(Signal), Detect increase/1(Signal), Detect increase2/1(Signal)
  Hold1/1("  ") -> Memory2/1
  Logical Operator/1 -> End of complete step/1
  Memory2/1 -> Logical Operator/2
  Detect increase2/1(Increase) -> Logical Operator/1
  Logical Operator1/1 -> Logical Operator2/3

== system MIL_Test/Validation Function/Feature extraction/Complete step detection/Step detection reset ==
  Step : Inport  OutDataType=sfix(16)  OutScaling=2^0
  Step response : Inport  Port=2  OutDataType=sfix(16)  OutScaling=2^0
  Active if signals constant for some specified time : Subsystem
  Logical Operator : Logic  AllPortsSameDT=off  OutDataTypeMode=boolean
  Memory : Memory
  Step detection : Subsystem  TreatAsAtomicUnit=on  mask(Feature extraction block){StepSize=10}
      mask prompts: StepSize "Minimum step size"
      mask help: Detect a step in the signal. The minimum step size is defined by the user.
      mask CallbackString:
      | if str2double(get_param(gcb,'StepSize')) <= 0
      |     error(['Minimum step size (' get_param(gcb,'StepSize') ') out of range. Please give a value greater than zero.']);
      | else
      |     set_param([gcb '/Min step size'],'Value',get_param(gcb,'StepSize'));
      | end
  R : Outport  OutDataType=sfix(16)  OutScaling=2^0
  wires:
  Logical Operator/1 -> R/1
  Step detection/1(Step) -> Logical Operator/2
  Step response/1 -> Active if signals constant for some specified time/1(Signal1)
  Memory/1 -> Logical Operator/1
  Active if signals constant for some specified time/1(Constant signals) -> Memory/1
  Step/1 -> Active if signals constant for some specified time/2(Signal 2), Step detection/1(Signal)

== system MIL_Test/Validation Function/Feature extraction/Detect constant/Relative tolerance ==
  sig : Inport  OutDataType=sfix(16)  OutScaling=2^0
  ref : Inport  Port=2  OutDataType=sfix(16)  OutScaling=2^0
  Abs : Abs
  Abs1 : Abs
  Add : Sum  Inputs=+-  OutDataType=sfix(16)  OutScaling=2^-10
  Divide1 : Product  Inputs=**/  OutDataType=sfix(16)  OutScaling=2^-10
  Max : Constant  Value=100  OutDataType=sfix(16)  OutScaling=2^0
  Relational Operator : RelationalOperator  Operator===  LogicOutDataTypeMode=boolean
  Relative Tolerance : Constant  OutDataType=sfix(16)  OutScaling=2^0
  sig == ref : Outport  OutDataType=sfix(16)  OutScaling=2^0
  wires:
  Abs1/1 -> Divide1/1
  Relational Operator/1 -> sig == ref/1
  Relative Tolerance/1 -> Divide1/2
  Max/1 -> Divide1/3
  Divide1/1 -> Relational Operator/2
  ref/1 -> Abs1/1, Add/2
  sig/1 -> Add/1
  Add/1 -> Abs/1
  Abs/1 -> Relational Operator/1

== system MIL_Test/Validation Function/Feature extraction/Linear relation/Relative tolerance ==
  sig : Inport  OutDataType=sfix(16)  OutScaling=2^0
  ref : Inport  Port=2  OutDataType=sfix(16)  OutScaling=2^0
  Abs : Abs
  Abs1 : Abs
  Add : Sum  Inputs=+-  OutDataType=sfix(16)  OutScaling=2^-10
  Divide1 : Product  Inputs=**/  OutDataType=sfix(16)  OutScaling=2^-10
  Max : Constant  Value=100  OutDataType=sfix(16)  OutScaling=2^0
  Relational Operator : RelationalOperator  Operator=<=  LogicOutDataTypeMode=boolean
  Relative Tolerance : Constant  Value=0.0001  OutDataType=sfix(16)  OutScaling=2^0
  sig == ref : Outport  OutDataType=sfix(16)  OutScaling=2^0
  wires:
  Abs1/1 -> Divide1/1
  Relational Operator/1 -> sig == ref/1
  Relative Tolerance/1 -> Divide1/2
  Max/1 -> Divide1/3
  Divide1/1 -> Relational Operator/2
  ref/1 -> Abs1/1, Add/2
  sig/1 -> Add/1
  Add/1 -> Abs/1
  Abs/1 -> Relational Operator/1

== system MIL_Test/Validation Function/Feature extraction/Signal value @ maximum/Local maximum ==
  Signal : Inport  OutDataType=sfix(16)  OutScaling=2^0
  Clock : Clock
      settings: Decimation=10
  Clock1 : Clock
      settings: Decimation=10
  Logical Operator : Logic  AllPortsSameDT=off  OutDataTypeMode=boolean
  Memory : Memory
  Memory1 : Memory
  Relational Operator : RelationalOperator  Operator=<  LogicOutDataTypeMode=boolean
  Relational Operator1 : RelationalOperator  Operator=>  LogicOutDataTypeMode=boolean
  Switch : Switch  Criteria=u2 > Threshold
  Switch1 : Switch  Criteria=u2 > Threshold
  Maximum : Outport  OutDataType=sfix(16)  OutScaling=2^0
  wires:
  Switch1/1 -> Relational Operator1/2
  Memory1/1 -> Switch1/1
  Clock1/1 -> Switch1/2
  Switch/1 -> Relational Operator1/1, Switch1/3, Memory1/1, Relational Operator/2
  Memory/1 -> Switch/1
  Clock/1 -> Switch/2
  Relational Operator/1 -> Logical Operator/1
  Relational Operator1/1 -> Logical Operator/2
  Logical Operator/1 -> Maximum/1
  Signal/1 -> Switch/3, Memory/1, Relational Operator/1

== system MIL_Test/Validation Function/Feature extraction/Step response characteristics/Step response characteristics extraction ==
  R : Inport  OutDataType=sfix(16)  OutScaling=2^0
  Step : Inport  Port=2  OutDataType=sfix(16)  OutScaling=2^0
  Step response : Inport  Port=3  OutDataType=sfix(16)  OutScaling=2^0
  Clock : Clock
      settings: Decimation=10
  Expected set point and step parameters : Subsystem  TreatAsAtomicUnit=on
  Extract maximum overshoot : Subsystem
  Extract rise time : Subsystem
  Extract settling time : Subsystem
  Extract steady state error : Subsystem
  Memory : Memory
  Static Gain : Constant  Value=0.8333  OutDataType=sfix(16)  OutScaling=2^0
  Step time : Subsystem  TreatAsAtomicUnit=on
  Rise time : Outport  DataType=double  OutDataType=sfix(16)  OutScaling=2^0
  Maximum overshoot : Outport  Port=2  DataType=double  OutDataType=sfix(16)  OutScaling=2^0
  Settling time : Outport  Port=3  DataType=double  OutDataType=sfix(16)  OutScaling=2^0
  Steady state error : Outport  Port=4  DataType=double  OutDataType=sfix(16)  OutScaling=2^0
  wires:
  Expected set point and step parameters/1(Step sign) -> Extract maximum overshoot/3(Step sign)
  Expected set point and step parameters/3(Response step size) -> Extract rise time/4(Response step size)
  Step response/1 -> Extract rise time/1(Step response), Extract maximum overshoot/1(Step response), Extract settling time/1(Step response), Extract steady state error/1(Step response)
  Step time/1(Time) -> Extract settling time/4(Step time)
  Expected set point and step parameters/2(Set point) -> Extract rise time/3(Set point), Extract settling time/2(Set point), Extract steady state error/2(Set point)
  Extract steady state error/1(ss error) -> Steady state error/1
  Memory/1 -> Expected set point and step parameters/1(Step/z)
  Clock/1 -> Step time/1(Clock)
  Step/1 -> Expected set point and step parameters/2(Step), Memory/1
  R/1 -> Extract settling time/3(Reset), Extract maximum overshoot/2(Reset), Extract rise time/2(Reset), Expected set point and step parameters/Trigger, Step time/Trigger
  Static Gain/1 -> Expected set point and step parameters/3(Static Gain)
  Extract settling time/1(Settling time) -> Settling time/1
  Extract maximum overshoot/1(Maximum overshoot) -> Maximum overshoot/1
  Extract rise time/1(Rise time) -> Rise time/1

== system MIL_Test/Validation Function/Feature extraction/Step response characteristics/Step response reset ==
  Step : Inport  OutDataType=sfix(16)  OutScaling=2^0
  Step response : Inport  Port=2  OutDataType=sfix(16)  OutScaling=2^0
  Active if signals constant for some specified time : Subsystem
  Logical Operator : Logic  AllPortsSameDT=off  OutDataTypeMode=boolean
  Memory : Memory
  Step detection : Subsystem  TreatAsAtomicUnit=on  mask(Feature extraction block){StepSize=1}
      mask prompts: StepSize "Minimum step size"
      mask help: Detect a step in the signal. The minimum step size is defined by the user.
      mask CallbackString:
      | if str2double(get_param(gcb,'StepSize')) <= 0
      |     error(['Minimum step size (' get_param(gcb,'StepSize') ') out of range. Please give a value greater than zero.']);
      | else
      |     set_param([gcb '/Min step size'],'Value',get_param(gcb,'StepSize'));
      | end
  R : Outport  OutDataType=sfix(16)  OutScaling=2^0
  wires:
  Logical Operator/1 -> R/1
  Step detection/1(Step) -> Logical Operator/2
  Step response/1 -> Active if signals constant for some specified time/1(Signal1)
  Memory/1 -> Logical Operator/1
  Active if signals constant for some specified time/1(Constant signals) -> Memory/1
  Step/1 -> Active if signals constant for some specified time/2(Signal 2), Step detection/1(Signal)

== system MIL_Test/Validation Function/Feature extraction/Step response characteristics/Step response trigger ==
  Steady state error : Inport  OutDataType=sfix(16)  OutScaling=2^0
  Step response : Inport  Port=2  OutDataType=sfix(16)  OutScaling=2^0
  Abs : Abs
  Active if signals constant for some specified time : Subsystem
  Compare To Constant : Subsystem  mask(Compare To Constant){relop=<=, const=0.5, LogicOutDataTypeMode=uint8, ZeroCross=off}
      mask prompts: relop "Operator:"; const "Constant value:"; LogicOutDataTypeMode "Output data type mode:"; ZeroCross "Enable zero crossing detection"
      mask help: Determine how a signal compares to a constant.
      mask init:
      | blkName = gcb;
      | 
      | if strcmp(get_param(gcbh,'LogicOutDataTypeMode'),'boolean')
      | 	setValue = 'Boolean';
      | else
      | 	setValue = 'Specify via dialog';
      | end
      | 
      | set_param([blkName,'/Compare'],'relop',relop, ...
      | 	'LogicOutDataTypeMode', setValue, 'ZeroCross', ZeroCross);
      | 
      | if length(const) == 1
      |  str = [relop,' ',num2str(double(const))];
      | else
      |   str = [relop,' C'];
      | end
      mask StyleString: popup(==|~=|<|<=|>=|>),edit,popup(uint8|boolean),checkbox
      mask Display: disp(str)
  Data Type Conversion : DataTypeConversion  OutDataType=sfix(16)  OutScaling=2^0
  Data Type Conversion1 : DataTypeConversion  OutDataType=sfix(16)  OutScaling=2^0
  Detect increase : Subsystem  TreatAsAtomicUnit=on
  Logical Operator : Logic  AllPortsSameDT=off  OutDataTypeMode=boolean  LogicDataType=double
  Rise time T : Outport  DataType=double  OutDataType=sfix(16)  OutScaling=2^0
  Overshoot T : Outport  Port=2  DataType=double  OutDataType=sfix(16)  OutScaling=2^0
  Settling time T : Outport  Port=3  DataType=double  OutDataType=sfix(16)  OutScaling=2^0
  Steady state error T : Outport  Port=4  DataType=double  OutDataType=sfix(16)  OutScaling=2^0
  wires:
  Logical Operator/1 -> Data Type Conversion/1
  Detect increase/1(Increase) -> Data Type Conversion1/1, Logical Operator/2
  Abs/1 -> Compare To Constant/1(u)
  Compare To Constant/1(y) -> Logical Operator/1
  Steady state error/1 -> Abs/1
  Step response/1 -> Active if signals constant for some specified time/1(Signal1), Active if signals constant for some specified time/2(Signal 2)
  Active if signals constant for some specified time/1(Constant signals) -> Detect increase/1(Signal)
  Data Type Conversion1/1 -> Steady state error T/1
  Data Type Conversion/1 -> Settling time T/1, Overshoot T/1, Rise time T/1
